simulink model "filter_1"  (R2014b)
settings: Solver=ode45  StartTime=0.0  StopTime=inf  RelTol=1e-3
libraries: commchan3 x2, dsparch4 x2, simulink x1
settings Model: Creator=Ben  LastModifiedBy=Ben

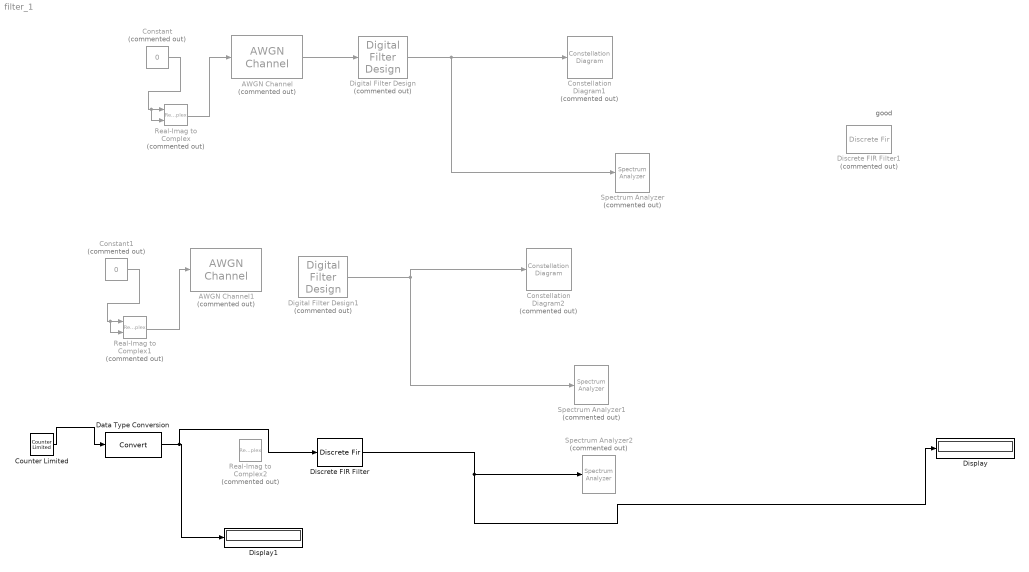
== system filter_1 ==
  note: good
  AWGN Channel : commchan3/AWGN Channel  Commented=on  InputProcessing=Columns as channels (frame based)  seed=67  noiseMode="Signal to noise ratio  (SNR)"  EbNodB=10  EsNodB=10  SNRdB=-10  bitsPerSym=1  Ps=1  Tsym=1  variance=1
  AWGN Channel1 : commchan3/AWGN Channel  Commented=on  InputProcessing=Columns as channels (frame based)  seed=67  noiseMode="Signal to noise ratio  (SNR)"  EbNodB=10  EsNodB=10  SNRdB=-10  bitsPerSym=1  Ps=1  Tsym=1  variance=1
  Constant : Constant  Commented=on  Value=0  SampleTime=1/250E6
  Constant1 : Constant  Commented=on  Value=0  SampleTime=1/125E3
  Constellation Diagram1 : ConstellationDiagram  Commented=on
  Constellation Diagram2 : ConstellationDiagram  Commented=on
  Counter Limited : simulink/Sources/Counter Limited  uplimit=15  tsamp=1/125E3
  Data Type Conversion : DataTypeConversion  RndMeth=Nearest
  Digital Filter Design : dsparch4/Digital Filter Design  Commented=on  mwdsp_browser_bugfix_var=off
  Digital Filter Design1 : dsparch4/Digital Filter Design  Commented=on  mwdsp_browser_bugfix_var=off
  Discrete FIR Filter : DiscreteFir  Coefficients=[.04 .05 .03]
  Discrete FIR Filter1 : DiscreteFir  Commented=on  Coefficients="[0.0075029723133660259 0.027258916482232186  0.055548646013161292  0.077030909792180635  0.077030909792180635  0.055548646013161292  0.027258916482232186  0.0075029723133660259 ]"
  Display : Display
  Display1 : Display
  Real-Imag to Complex : RealImagToComplex  Commented=on
  Real-Imag to Complex1 : RealImagToComplex  Commented=on
  Real-Imag to Complex2 : RealImagToComplex  Commented=on
  Spectrum Analyzer : SpectrumAnalyzer  Commented=on
  Spectrum Analyzer1 : SpectrumAnalyzer  Commented=on
  Spectrum Analyzer2 : SpectrumAnalyzer  Commented=on
  wires:
  AWGN Channel/1 -> Digital Filter Design/1
  Constant/1 -> Real-Imag to Complex/2, Real-Imag to Complex/1
  Real-Imag to Complex/1 -> AWGN Channel/1
  Digital Filter Design/1 -> Spectrum Analyzer/1, Constellation Diagram1/1
  Constant1/1 -> Real-Imag to Complex1/2, Real-Imag to Complex1/1
  Real-Imag to Complex1/1 -> AWGN Channel1/1
  Digital Filter Design1/1 -> Constellation Diagram2/1, Spectrum Analyzer1/1
  Discrete FIR Filter/1 -> Spectrum Analyzer2/1, Display/1
  Counter Limited/1 -> Data Type Conversion/1
  Data Type Conversion/1 -> Discrete FIR Filter/1, Display1/1
